simulink model "pmsm_comparison"  (R2022b)
settings: Solver=FixedStepAuto  StartTime=0.0  StopTime=simParam.stopTime  FixedStep=simParam.maxStep  MaxStep=simParam.maxStep  RelTol=1e-3
values from neighbouring files (symbols this model uses):
  b = 0.01    [control_pmsm.m]
  J = 0.1    [control_pmsm.m]
  lambdaM = 0.14    [control_pmsm.m]
  Ld = 0.9    [control_pmsm.m]
  linear =     [linearSystem.mat]
  Lq = 0.9    [control_pmsm.m]
  N = 18    [control_pmsm.m]
  opPoint =     [linearSystem.mat]
  Rs = 1.3    [control_pmsm.m]
undefined symbols (not defined in the file or in its folder): aug, simParam, X_i
settings Model: Creator=kaike  LastModifiedBy=kaike

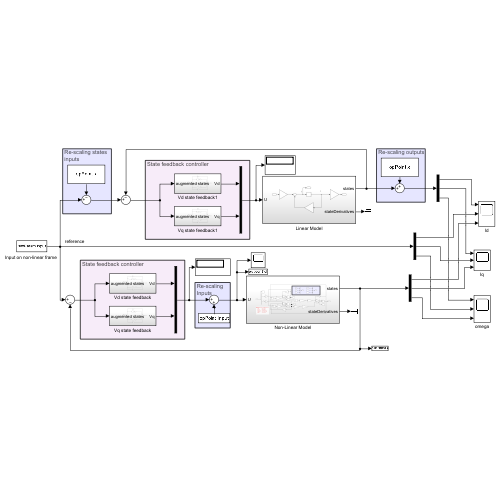
[thumbnail: Simulink's stored preview of the top-level diagram]
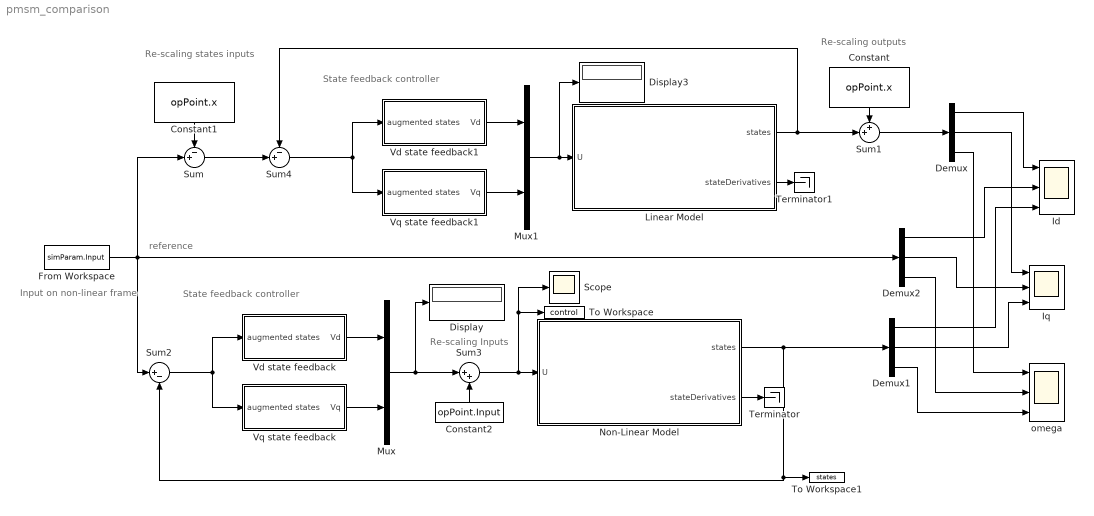
== system pmsm_comparison ==
  note: Re-scaling
      | Inputs
  note: Input on non-linear frame
  note: reference
  note: Re-scaling outputs
  note: State feedback controller
  note: Re-scaling states
      | inputs
  note: State feedback controller
  Constant : Constant  Value=opPoint.x
  Constant1 : Constant  Value=opPoint.x
  Constant2 : Constant  Value=opPoint.Input
  Demux : Demux  Outputs=3
  Demux1 : Demux  Outputs=3
  Demux2 : Demux  Outputs=3
  Display : Display
  Display3 : Display
  From Workspace : FromWorkspace  VariableName=simParam.Input  OutputAfterFinalValue=Holding final value
  Id : Scope  NumInputPorts=3
  Iq : Scope  NumInputPorts=3
  Linear Model : Subsystem
  Mux : Mux  Inputs=2
  Mux1 : Mux  Inputs=2
  "Non-Linear Model " : Subsystem
  Scope : Scope
  Sum : Sum  Inputs=-+|
  Sum1 : Sum  Inputs=++|
  Sum2 : Sum  Inputs=|+-
  Sum3 : Sum  Inputs=|++
  Sum4 : Sum  Inputs=-+|
  Terminator : Terminator
  Terminator1 : Terminator
  To Workspace : ToWorkspace  VariableName=control  SampleTime=-1
  To Workspace1 : ToWorkspace  VariableName=states  SampleTime=-1
  Vd state feedback : Subsystem
  Vd state feedback1 : Subsystem
  Vq state feedback : Subsystem
  Vq state feedback1 : Subsystem
  omega : Scope  NumInputPorts=3
  wires:
  "Non-Linear Model "/2(stateDerivatives) -> Terminator/1
  Constant1/1 -> Sum/1
  Constant/1 -> Sum1/1
  Vd state feedback/1(Vd) -> Mux/1
  Vq state feedback/1(Vq) -> Mux/2
  Sum2/1 -> Vq state feedback/1(augmented states), Vd state feedback/1(augmented states)
  From Workspace/1 -> Sum2/1, Sum/2, Demux2/1
  Sum1/1 -> Demux/1
  Demux1/3 -> omega/3
  Demux/3 -> omega/1
  Demux/1 -> Id/1
  Demux1/1 -> Id/3
  Demux2/1 -> Id/2
  Demux2/3 -> omega/2
  Demux/2 -> Iq/1
  Demux2/2 -> Iq/2
  Demux1/2 -> Iq/3
  "Non-Linear Model "/1(states) -> Demux1/1, Sum2/2, To Workspace1/1
  Constant2/1 -> Sum3/2
  Sum3/1 -> To Workspace/1, Scope/1, "Non-Linear Model "/1(U)
  Mux/1 -> Sum3/1, Display/1
  Vq state feedback1/1(Vq) -> Mux1/2
  Sum4/1 -> Vq state feedback1/1(augmented states), Vd state feedback1/1(augmented states)
  Vd state feedback1/1(Vd) -> Mux1/1
  Mux1/1 -> Display3/1, Linear Model/1(U)
  Sum/1 -> Sum4/2
  Linear Model/1(states) -> Sum1/2, Sum4/1
  Linear Model/2(stateDerivatives) -> Terminator1/1

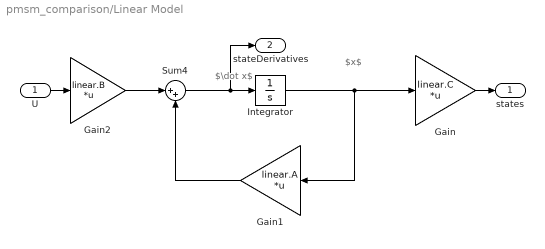
== system pmsm_comparison/Linear Model ==
  note: $\dot x$
  note: $x$
  U : Inport
  Gain : Gain  Gain=linear.C  Multiplication=Matrix(K*u)
  Gain1 : Gain  Gain=linear.A  Multiplication=Matrix(K*u)
  Gain2 : Gain  Gain=linear.B  Multiplication=Matrix(K*u)
  Integrator : Integrator
  Sum4 : Sum  Inputs=|++
  states : Outport
  stateDerivatives : Outport  Port=2
  wires:
  Gain1/1 -> Sum4/2
  Gain/1 -> states/1
  Integrator/1 -> Gain1/1, Gain/1
  Sum4/1 -> stateDerivatives/1, Integrator/1
  Gain2/1 -> Sum4/1
  U/1 -> Gain2/1

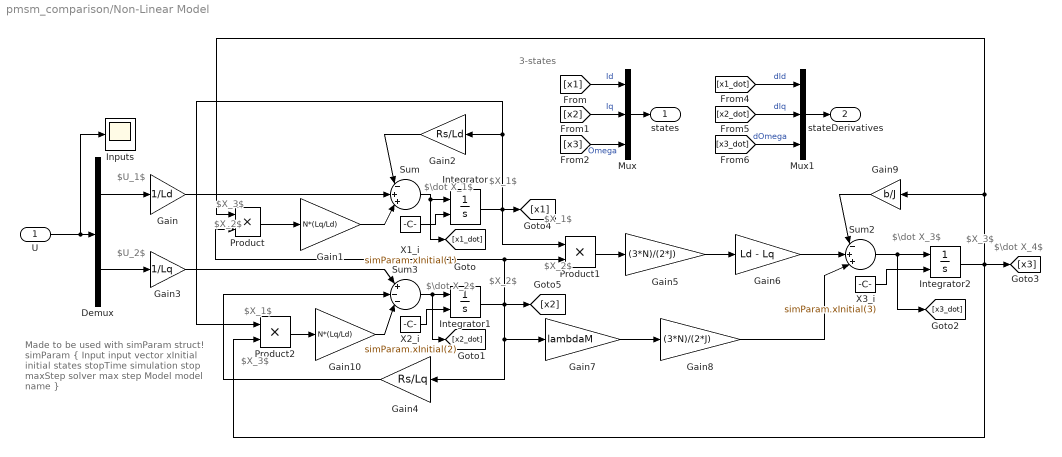
== system pmsm_comparison/Non-Linear Model  ==
  note: $U_1$
  note: $X_3$
  note: $\dot X_1$
  note: $\dot X_4$
  note: $\dot X_2$
  note: $X_1$
  note: $X_2$
  note: $\dot X_3$
  note: Made to be used with simParam struct!
      | simParam {
      | Input input vector
      | xInitial initial states
      | stopTime simulation stop
      | maxStep solver max step
      | Model model name
      | }
  note: $X_3$
  note: $X_1$
  note: $X_1$
  note: $X_3$
  note: $X_2$
  note: $X_2$
  note: 3-states
  note: $U_2$
  U : Inport
  Demux : Demux  Outputs=2
  Gain : Gain  Gain=1/Ld
  Gain1 : Gain  Gain=N*(Lq/Ld)
  Gain10 : Gain  Gain=N*(Lq/Ld)
  Gain2 : Gain  Gain=Rs/Ld
  Gain3 : Gain  Gain=1/Lq
  Gain4 : Gain  Gain=Rs/Lq
  Gain5 : Gain  Gain=(3*N)/(2*J)
  Gain6 : Gain  Gain=Ld - Lq
  Gain7 : Gain  Gain=lambdaM
  Gain8 : Gain  Gain=(3*N)/(2*J)
  Gain9 : Gain  Gain=b/J
  Inputs : Scope
  Integrator : Integrator  InitialConditionSource=external  InitialCondition=simParam.X_initial(3)  ContinuousStateAttributes='Id'
  Integrator1 : Integrator  InitialConditionSource=external  InitialCondition=X_i(2)  ContinuousStateAttributes='Iq'
  Integrator2 : Integrator  InitialConditionSource=external  InitialCondition=10  ContinuousStateAttributes='omega'
  Mux : Mux  Inputs=3
  Mux1 : Mux  Inputs=3
  Product : Product
  Product1 : Product
  Product2 : Product
  Sum : Sum  Inputs=|-++|
  Sum2 : Sum  Inputs=|-++|
  Sum3 : Sum  Inputs=|+--|
  X1_i : Constant  Value=simParam.xInitial(1)  VectorParams1D=off
  X2_i : Constant  Value=simParam.xInitial(2)
  X3_i : Constant  Value=simParam.xInitial(3)
  states : Outport
  stateDerivatives : Outport  Port=2
  wires:
  Gain6/1 -> Sum2/2
  Mux1/1 -> stateDerivatives/1
  Product1/1 -> Gain5/1
  Gain1/1 -> Sum/3
  Integrator2/1 -> [x3], Product2/2, Gain9/1, Product/1
  Gain3/1 -> Sum3/1
  Mux/1 -> states/1
  Gain9/1 -> Sum2/1
  Gain2/1 -> Sum/1
  Sum3/1 -> [x2_dot], Integrator1/1
  Sum2/1 -> [x3_dot], Integrator2/1
  Gain4/1 -> Sum3/2
  Integrator1/1 -> [x2], Product/2, Product1/2, Gain4/1, Gain7/1
  [x3_dot] -> Mux1/3  "dOmega"
  U/1 -> Inputs/1, Demux/1
  [x1] -> Mux/1  "Id"
  X1_i/1 -> Integrator/2
  Product2/1 -> Gain10/1
  X3_i/1 -> Integrator2/2
  Gain8/1 -> Sum2/3
  [x2] -> Mux/2  "Iq"
  Sum/1 -> [x1_dot], Integrator/1
  [x2_dot] -> Mux1/2  "dIq"
  Demux/1 -> Gain/1
  Gain10/1 -> Sum3/3
  Product/1 -> Gain1/1
  X2_i/1 -> Integrator1/2
  Demux/2 -> Gain3/1
  Gain7/1 -> Gain8/1
  Integrator/1 -> [x1], Product2/1, Gain2/1, Product1/1
  [x1_dot] -> Mux1/1  "dId"
  [x3] -> Mux/3  "Omega"
  Gain/1 -> Sum/2
  Gain5/1 -> Gain6/1

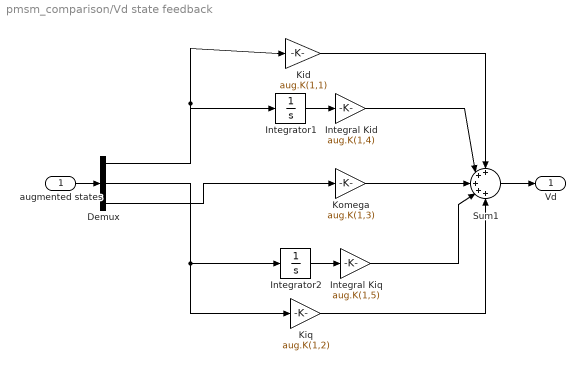
== system pmsm_comparison/Vd state feedback ==
  augmented states : Inport
  Demux : Demux  Outputs=3
  Integral Kid : Gain  Gain=aug.K(1,4)
  Integral Kiq : Gain  Gain=aug.K(1,5)
  Integrator1 : Integrator
  Integrator2 : Integrator
  Kid : Gain  Gain=aug.K(1,1)
  Kiq : Gain  Gain=aug.K(1,2)
  Komega : Gain  Gain=aug.K(1,3)
  Sum1 : Sum  Inputs=+++++
  Vd : Outport
  wires:
  augmented states/1 -> Demux/1
  Integrator1/1 -> Integral Kid/1
  Sum1/1 -> Vd/1
  Integrator2/1 -> Integral Kiq/1
  Demux/1 -> Kid/1, Integrator1/1
  Integral Kid/1 -> Sum1/2
  Kid/1 -> Sum1/1
  Demux/3 -> Komega/1
  Komega/1 -> Sum1/3
  Demux/2 -> Kiq/1, Integrator2/1
  Integral Kiq/1 -> Sum1/4
  Kiq/1 -> Sum1/5

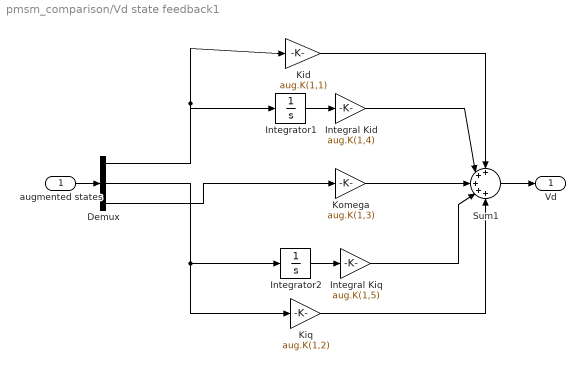
== system pmsm_comparison/Vd state feedback1 ==
  augmented states : Inport
  Demux : Demux  Outputs=3
  Integral Kid : Gain  Gain=aug.K(1,4)
  Integral Kiq : Gain  Gain=aug.K(1,5)
  Integrator1 : Integrator
  Integrator2 : Integrator
  Kid : Gain  Gain=aug.K(1,1)
  Kiq : Gain  Gain=aug.K(1,2)
  Komega : Gain  Gain=aug.K(1,3)
  Sum1 : Sum  Inputs=+++++
  Vd : Outport
  wires:
  augmented states/1 -> Demux/1
  Integrator1/1 -> Integral Kid/1
  Sum1/1 -> Vd/1
  Integrator2/1 -> Integral Kiq/1
  Demux/1 -> Kid/1, Integrator1/1
  Integral Kid/1 -> Sum1/2
  Kid/1 -> Sum1/1
  Demux/3 -> Komega/1
  Komega/1 -> Sum1/3
  Demux/2 -> Kiq/1, Integrator2/1
  Integral Kiq/1 -> Sum1/4
  Kiq/1 -> Sum1/5

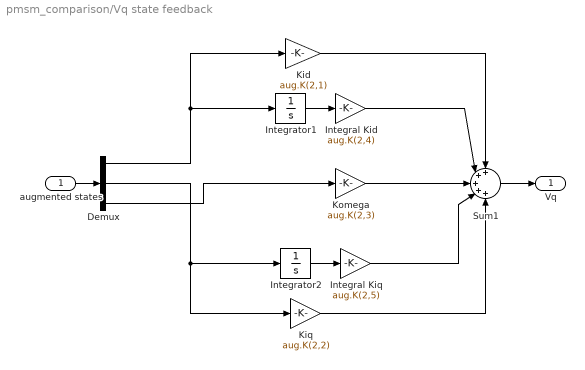
== system pmsm_comparison/Vq state feedback ==
  augmented states : Inport
  Demux : Demux  Outputs=3
  Integral Kid : Gain  Gain=aug.K(2,4)
  Integral Kiq : Gain  Gain=aug.K(2,5)
  Integrator1 : Integrator
  Integrator2 : Integrator
  Kid : Gain  Gain=aug.K(2,1)
  Kiq : Gain  Gain=aug.K(2,2)
  Komega : Gain  Gain=aug.K(2,3)
  Sum1 : Sum  Inputs=+++++
  Vq : Outport
  wires:
  augmented states/1 -> Demux/1
  Integrator1/1 -> Integral Kid/1
  Sum1/1 -> Vq/1
  Integrator2/1 -> Integral Kiq/1
  Demux/1 -> Kid/1, Integrator1/1
  Integral Kid/1 -> Sum1/2
  Kid/1 -> Sum1/1
  Demux/3 -> Komega/1
  Komega/1 -> Sum1/3
  Demux/2 -> Kiq/1, Integrator2/1
  Integral Kiq/1 -> Sum1/4
  Kiq/1 -> Sum1/5

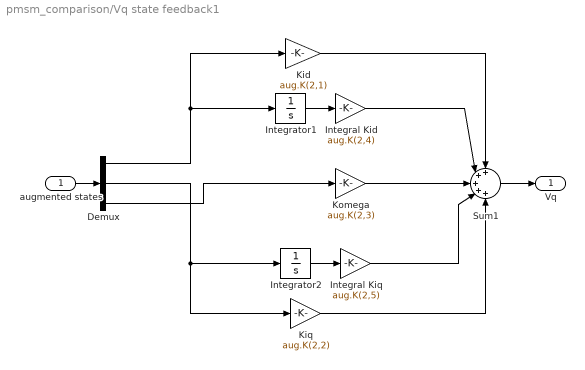
== system pmsm_comparison/Vq state feedback1 ==
  augmented states : Inport
  Demux : Demux  Outputs=3
  Integral Kid : Gain  Gain=aug.K(2,4)
  Integral Kiq : Gain  Gain=aug.K(2,5)
  Integrator1 : Integrator
  Integrator2 : Integrator
  Kid : Gain  Gain=aug.K(2,1)
  Kiq : Gain  Gain=aug.K(2,2)
  Komega : Gain  Gain=aug.K(2,3)
  Sum1 : Sum  Inputs=+++++
  Vq : Outport
  wires:
  augmented states/1 -> Demux/1
  Integrator1/1 -> Integral Kid/1
  Sum1/1 -> Vq/1
  Integrator2/1 -> Integral Kiq/1
  Demux/1 -> Kid/1, Integrator1/1
  Integral Kid/1 -> Sum1/2
  Kid/1 -> Sum1/1
  Demux/3 -> Komega/1
  Komega/1 -> Sum1/3
  Demux/2 -> Kiq/1, Integrator2/1
  Integral Kiq/1 -> Sum1/4
  Kiq/1 -> Sum1/5
